simulink model "Q3"  (R2018a)
settings: Solver=VariableStepAuto  StartTime=0.0  StopTime=1e5  RelTol=1e-3
undefined symbols (not defined in the file or in its folder): m, n
settings Model: Creator=Mohamed Saber  LastModifiedBy=Mohamed Saber

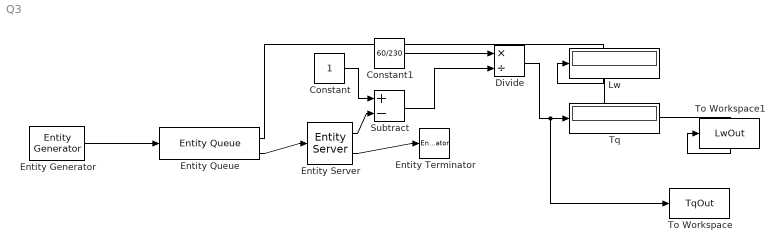
== system Q3 ==
  Constant : Constant
  Constant1 : Constant  Value=60/230
  Divide : Product  Inputs=*/
  Entity Generator : EntityGenerator  OutputPortMessageModes=m  TimeSource=MATLAB action  IntergenerationTimeAction=|  GenerateAction=|  AttributeName=ClassA  EntityType=Structured  EntityTypeName=Entity
      IntergenerationTimeAction=|
      | dt = rand(1,1);
      | persistent rngInit;
      | if isempty(rngInit)
      |     seed = 12345;
      |     rng(seed);
      |     rngInit = true;
      | end
      | 
      | % Pattern: Exponential distribution
      | mu = 60/220;
      | dt = -mu * log(1 - rand());
      GenerateAction=|
      | persistent rngInit;
      | if isempty(rngInit)
      |     seed = 15318;
      |     rng(seed);
      |     rngInit = true;
      | end
      | 
      | % Pattern: Arbitrary discrete distribution
      | % V: Value vector
      | % P: Probability vector
      | V = [1 2];
      | P = [0.2 0.8];
      | entity.ClassA = randsample(V, 1, true, P);
  Entity Queue : EntityQueue  InputPortMessageModes=m  OutputPortMessageModes=n,m  Capacity=inf  PrioritySource=ClassA  AverageQueueLength=on
      settings: OutputPortMap=o3,o5
  Entity Server : EntityServer  InputPortMessageModes=m  OutputPortMessageModes=n,m  Capacity=c  ServiceTimeSource=MATLAB action  ServiceTimeValue=60/220  ServiceTimeAttributeName=ClassA  ServiceTimeAction=|  Utilization=on
      | dt = rand(1,1);
      | persistent rngInit;
      | if isempty(rngInit)
      |     seed = 845889;
      |     rng(seed);
      |     rngInit = true;
      | end
      | 
      | % Pattern: Exponential distribution
      | mu = 60/230;
      | dt = -mu * log(1 - rand());
      settings: OutputPortMap=o5,o9
  Entity Terminator : EntityTerminator  InputPortMessageModes=m
  Lw : Display
  Subtract : Sum  Inputs=+-
  To Workspace : ToWorkspace  VariableName=TqOut  SampleTime=-1
      settings: Save2DSignal=2-D array (concatenate along first dimension)
  To Workspace1 : ToWorkspace  VariableName=LwOut  SampleTime=-1
      settings: Save2DSignal=2-D array (concatenate along first dimension)
  Tq : Display
  wires:
  Entity Server/1 -> Subtract/2
  Constant1/1 -> Divide/1
  Constant/1 -> Subtract/1
  Entity Server/2 -> Entity Terminator/1
  Entity Queue/1 -> To Workspace1/1, Lw/1
  Divide/1 -> To Workspace/1, Tq/1
  Entity Generator/1 -> Entity Queue/1
  Entity Queue/2 -> Entity Server/1
  Subtract/1 -> Divide/2
